simulink model "sl_pmsm"  (R2023b)
settings: Solver=VariableStepAuto  StartTime=0.0  StopTime=3  FixedStep=0.02  MaxStep=0.02  RelTol=1e-3
InitFcn:
  | init
values from neighbouring files (symbols this model uses):
  pa = block.DialogPrm(1).Data    [Animation.m]    (also in Saddle_Wave.m; current_controller.m; flux_dynamic.m; mechanical_equation.m)
libraries: spsVoltageMeasurementLib x9, simulink x4, spsSeriesRLCBranchLib x3, spsDCVoltageSourceLib x2, slpidlib x1, SignalEditorBlockLib x1, spsGroundLib x1, spsUniversalBridgeLib x1, spspowerguiLib x1
settings Model: Creator=PC  LastModifiedBy=PC

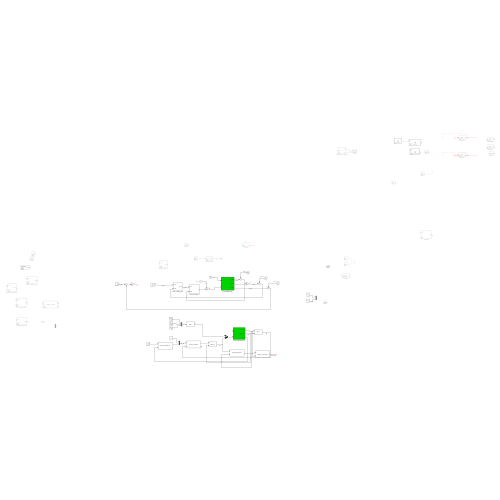
[thumbnail: Simulink's stored preview of the top-level diagram]
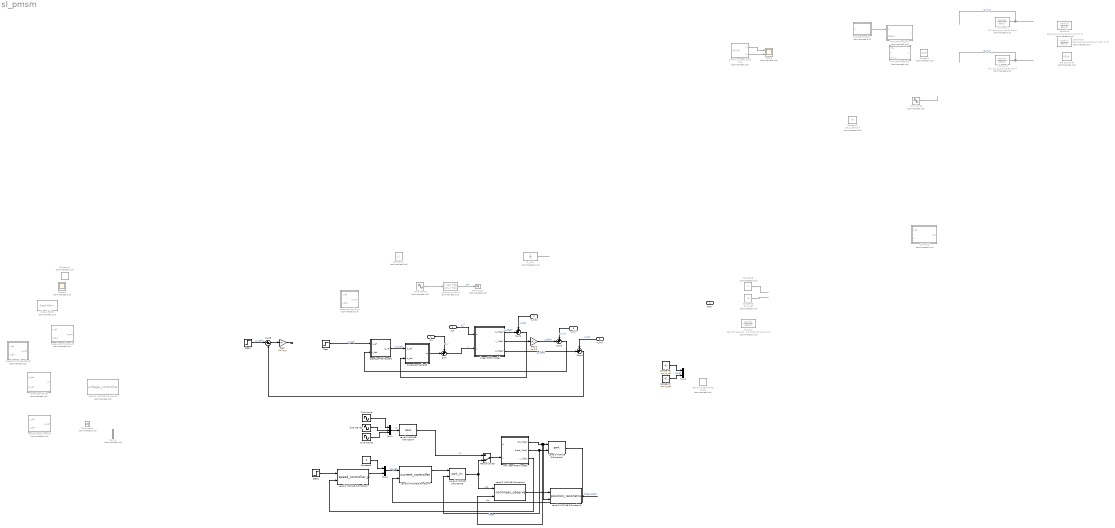
== system sl_pmsm ==
  d_v : Inport
  "n_{iq}" : Inport  Port=2
  "n_{v}" : Inport  Port=3
  d_T : Inport  Port=4
  "n_{p}" : Inport  Port=5
  Band-Limited White Noise : simulink/Sources/Band-Limited White Noise  Commented=on  Cov=[0.1]  Ts=0.1  seed=[23341]
  Constant : Constant  Commented=on  Value=pa.P
  Constant1 : Constant  Commented=on  Value=pa.iq_ref*pa.R
  Constant2 : Constant  Commented=on  Value=0.1
  Constant3 : Constant  Value=0
  Constant4 : Constant  Commented=on  Value=pa.v_ref
  Constant5 : Constant  Commented=on  Value=0
  Constant6 : Constant  Value=pa.vd_ref
  Constant7 : Constant  Value=pa.vq_ref
  Constant8 : Constant  Commented=on  Value=pa.iq_ref
  Demux : Demux  Commented=on  Outputs=2
  G_iq2w : TransferFcn  Commented=on  Denominator=[1 0]
  G_uq2w : TransferFcn  Commented=on  Numerator=[pa.Kt]  Denominator=[pa.Lq*pa.J pa.B*pa.Lq+pa.J*pa.R pa.B*pa.R+pa.Kt*pa.P/2*pa.phi_m]
  Gain : Gain  Gain=pa.Kp_p
  Gain1 : Gain  Gain=pa.P/2
  Id dynamic : TransferFcn  Commented=on  Denominator=[pa.Ls_d_H pa.Rs_Ohm]
  Iq dynamic : TransferFcn  Commented=on  Denominator=[pa.Ls_q_H pa.Rs_Ohm]
  Level-2 MATLAB S-Function1 : M-S-Function  FunctionName=speed_controller_pi  Parameters=pa
  Level-2 MATLAB S-Function2 : M-S-Function  Commented=on  FunctionName=voltage_controller  Parameters=pa
  Level-2 MATLAB S-Function3 : M-S-Function  FunctionName=nonlinear_observer  Parameters=pa
  Level-2 MATLAB S-Function4 : M-S-Function  FunctionName=current_controller  Parameters=pa
  Level-2 MATLAB S-Function5 : M-S-Function  FunctionName=park  Parameters=pa
  Level-2 MATLAB S-Function6 : M-S-Function  FunctionName=position_reconstruct  Parameters=pa
  Level-2 MATLAB S-Function7 : M-S-Function  FunctionName=clark  Parameters=pa
  Level-2 MATLAB S-Function8 : M-S-Function  FunctionName=park_inv  Parameters=pa
  MATLAB Function : MATLAB Function  Commented=on  TreatAsAtomicUnit=on
  MATLAB Function1 : MATLAB Function  Commented=on  TreatAsAtomicUnit=on
  MATLAB Function2 : MATLAB Function  Commented=on  TreatAsAtomicUnit=on
  Manual Switch : ManualSwitch  CurrentSetting=0
  Mux1 : Mux  Inputs=3
  Mux2 : Mux  Inputs=2
  Mux3 : Mux  Inputs=2
  PID Controller : slpidlib/PID Controller  Commented=on  Controller=PID  Form=Parallel  TimeDomain=Continuous-time  UseExternalTs=off  SampleTime=-1  IntegratorMethod=Forward Euler  FilterMethod=Forward Euler  ControllerParametersSource=internal  P=1  I=1  UseKiTs=off  D=0  N=100  UseFilter=on  TunerSelectOption=Transfer Function Based (PID Tuner App)  InitialConditionSource=internal  InitialConditionForIntegrator=0  InitialConditionForFilter=0  DifferentiatorICPrevScaledInput=0  ExternalReset=none  TrackingMode=off  Kt=1  LimitOutput=off  SatLimitsSource=internal  UpperSaturationLimit=inf  LowerSaturationLimit=-inf  LinearizeAsGain=on  AntiWindupMode=none  Kb=1  LimitIntegrator=off  UpperIntegratorSaturationLimit=inf  LowerIntegratorSaturationLimit=-inf  POutMin=[]  POutMax=[]  IOutMin=[]  IOutMax=[]  DOutMin=[]  DOutMax=[]  NOutMin=[]  NOutMax=[]  SumOutMin=[]  SumOutMax=[]  SaturationOutMin=[]  SaturationOutMax=[]  PParamMin=[]  PParamMax=[]  IParamMin=[]  IParamMax=[]  DParamMin=[]  DParamMax=[]  NParamMin=[]  NParamMax=[]  KbParamMin=[]  KbParamMax=[]  KtParamMin=[]  KtParamMax=[]  KbOutMin=[]  KbOutMax=[]  KtOutMin=[]  KtOutMax=[]  IntegratorOutMin=[]  IntegratorOutMax=[]  FilterOutMin=[]  FilterOutMax=[]  SumI1OutMin=[]  SumI1OutMax=[]  SumI2OutMin=[]  SumI2OutMax=[]  SumI3OutMin=[]  SumI3OutMax=[]  SumI4OutMin=[]  SumI4OutMax=[]  SumDOutMin=[]  SumDOutMax=[]  DifferentiatorOutMin=[]  DifferentiatorOutMax=[]  FilterDiffOutCoefMin=[]  FilterDiffOutCoefMax=[]  ReciprocalOutMin=[]  ReciprocalOutMax=[]  SumDenOutMin=[]  SumDenOutMax=[]  SumNumOutMin=[]  SumNumOutMax=[]  DivideOutMin=[]  DivideOutMax=[]  UdiffTsProdOutMin=[]  UdiffTsProdOutMax=[]  NTsProdOutMin=[]  NTsProdOutMax=[]  UintegralTsProdOutMin=[]  UintegralTsProdOutMax=[]  UngainTsProdOutMin=[]  UngainTsProdOutMax=[]  ClampingZeroOutDataTypeStr=Inherit: Inherit via back propagation  ClampingZeroOutMin=[]  ClampingZeroOutMax=[]  FilterDenConstantOutDataTypeStr=Inherit: Inherit via back propagation  FilterDenConstantOutMin=[]  FilterDenConstantOutMax=[]  PCopyOutDataTypeStr=Inherit: Inherit via back propagation  PCopyOutMin=[]  PCopyOutMax=[]  NCopyOutDataTypeStr=Inherit: Inherit via back propagation  NCopyOutMin=[]  NCopyOutMax=[]  IntegratorContinuousStateAttributes=''  IntegratorStateMustResolveToSignalObject=off  IntegratorRTWStateStorageClass=Auto  FilterContinuousStateAttributes=''  FilterStateMustResolveToSignalObject=off  FilterRTWStateStorageClass=Auto  ParallelPVariant=InternalParameters  IdealPVariant=Disabled  IVariant=InternalParameters  DVariant=InternalParameters  IntegratorVariant=Continuous  SatVariant=Disabled  AWVariant=Passthrough  PCopyVariant=Disabled  TRVariant=Disabled  FdbkBlocksVariant=Forward  IdealPFdbkVariant=Disabled  SatFdbkVariant=Disabled  DerivativeFilterVariant=ContFilter  NVariant=InternalParameters  NCopyVariant=Disabled  FilterICVariant=InternalICsFilter  IntegratorICVariant=InternalICs  ExternalResetVariant=Disabled  TRSumVariant=Passthrough  SumFdbkVariant=Disabled  SumVariant=Sum_PID  TsampFilterVariant=InternalTs  TsampNgainVariant=Passthrough  TsampIntegralVariant=Disabled_SignalSpec  ExternalSaturationOutDataTypeStr=Inherit: Same as second input
  Scope : Scope  Commented=on  NumInputPorts=2
  Scope1 : Scope  Commented=on
  Signal Editor : SignalEditorBlockLib/Signal Editor  Commented=on  FileName=ramp.mat  ActiveScenario=Scenario  ActiveSignal=Signal 1  IsBus=off  OutputBusObjectStr=Bus: BusObject  SampleTime=0  Interpolate=off  ZeroCross=off  OutputAfterFinalValue=Holding final value  Unit=inherit  PreserveSignalName=on  ApplySigPropsToAllScenarios=on  ApplySigPropsToAllSignals=off
  Sine Wave : Sin  Frequency=50*2*pi  SampleTime=0
  Sine Wave1 : Sin  Frequency=50*2*pi  Phase=-2*pi/3  SampleTime=0
  Sine Wave2 : Sin  Frequency=50*2*pi  Phase=2*pi/3  SampleTime=0
  Sine Wave3 : Sin  Commented=on  Amplitude=1.0  Frequency=1*2*pi  SampleTime=0
  Sine Wave4 : Sin  Commented=on  Frequency=50*2*pi  Phase=-pi/2  SampleTime=0
  Step : Step  After=pa.v_ref  SampleTime=0
  Step1 : Step  After=pa.v_ref  SampleTime=0
  Step2 : Step  After=pa.p_vef  SampleTime=0
  Sum{,1..2,4} (4 alike) : Sum  Inputs=++|
  Sum3 : Sum  Inputs=|+-
  Terminator : Terminator  Commented=on
  Terminator1 : Terminator  Commented=on
  controller : TransferFcn  Commented=on  Numerator=[pa.Kp_Iq pa.Kp_Iq*pa.Ki_Iq]  Denominator=[1 0]
  controller1 : TransferFcn  Commented=on  Numerator=[pa.Kp_Id pa.Kp_Id*pa.Ki_Id]  Denominator=[1 0]
  controller_polynomial : Subsystem  Commented=on
  current_controller : Subsystem  Commented=on
  current_controller_tf : Subsystem
  dq model : Subsystem  Commented=on
  linear PMSM model : Subsystem
  nonlinear PMSM model : Subsystem
  simplify current close loop : Subsystem  Commented=on
  speed_controller_adrc : Subsystem
  speed_controller_adrc_tf : Subsystem  Commented=on
  speed_controller_pi : Subsystem  Commented=on
  speed_controller_pi_tf : Subsystem  Commented=on
  velocity dynamic : StateSpace  Commented=on  A=-0.5  B=1058  D=0  InitialCondition=0
  error : Outport
  wires:
  Iq dynamic/1 -> ?  "Iq_in_A"
  Id dynamic/1 -> ?  "Id_in_A"
  ? -> Id dynamic/1
  Step1/1 -> Level-2 MATLAB S-Function1/1
  ? -> Iq dynamic/1
  MATLAB Function/1(y) -> MATLAB Function1/1(u)
  Sine Wave/1 -> Mux1/1
  Sine Wave1/1 -> Mux1/2
  Sine Wave2/1 -> Mux1/3
  Mux1/1 -> Level-2 MATLAB S-Function7/1  "v1"
  Sine Wave4/1 -> ?
  Level-2 MATLAB S-Function7/1 -> Manual Switch/1  "v2"
  simplify current close loop/1(id) -> Scope/1
  simplify current close loop/2(iq) -> Scope/2
  Sine Wave3/1 -> velocity dynamic/1
  velocity dynamic/1 -> Terminator/1  "v_ol"
  Constant7/1 -> Mux2/2  "vq_ref"
  Constant6/1 -> Mux2/1
  current_controller_tf/1(uq) -> Sum/2
  d_v/1 -> Sum/1  "d_v"
  "n_{v}"/1 -> Sum2/1  "n_{v}"
  speed_controller_adrc/1(iq_ref) -> current_controller_tf/1(iq_ref)  "iq_{ref}"
  Constant8/1 -> ?
  Constant5/1 -> ?
  Constant3/1 -> Mux3/1
  Mux3/1 -> Level-2 MATLAB S-Function4/1  "idq_ref"
  Level-2 MATLAB S-Function1/1 -> Mux3/2
  Step2/1 -> Sum3/1  "p_{ref}"
  Sum3/1 -> Gain/1
  "n_{iq}"/1 -> Sum1/1  "n_{iq}"
  Sum1/1 -> current_controller_tf/2(iq_fed)
  d_T/1 -> linear PMSM model/1(d)  "d_T"
  Sum/1 -> linear PMSM model/2(u)  "u"
  linear PMSM model/1("iq_{fed}") -> Sum1/2  "iq_{fed}"
  linear PMSM model/2("v_{fed}") -> Gain1/1
  Manual Switch/1 -> nonlinear PMSM model/2(u)
  linear PMSM model/3("p_{fed}") -> Sum4/2  "p_{fed}"
  "n_{p}"/1 -> Sum4/1  "n_{p}"
  Step/1 -> speed_controller_adrc/1(v_ref)  "v_{ref}"
  Sum2/1 -> speed_controller_adrc/2(v_fed)
  Sum4/1 -> Sum3/2
  Gain/1 -> ?
  Gain1/1 -> Sum2/2  "v_{fed}"
  G_iq2w/1 -> ?
  nonlinear PMSM model/1("Iab_{fed}") -> Level-2 MATLAB S-Function6/2, Level-2 MATLAB S-Function5/1, Level-2 MATLAB S-Function3/2
  nonlinear PMSM model/2("theta_{fed}") -> Level-2 MATLAB S-Function8/2, Level-2 MATLAB S-Function5/2  "theta"
  Level-2 MATLAB S-Function5/1 -> Level-2 MATLAB S-Function4/2  "idq"
  nonlinear PMSM model/3("v_{fed}") -> Level-2 MATLAB S-Function1/2
  Level-2 MATLAB S-Function4/1 -> Level-2 MATLAB S-Function8/1
  Level-2 MATLAB S-Function8/1 -> Manual Switch/2, Level-2 MATLAB S-Function3/1  "vab"
  Level-2 MATLAB S-Function3/1 -> Level-2 MATLAB S-Function6/1
  Level-2 MATLAB S-Function6/1 -> ?  "theta_{hat}"

== system sl_pmsm/controller_polynomial ==
  v_ref : Inport
  v_fed : Inport  Port=2
  C_polynomial : TransferFcn  Numerator=[1 1]  Denominator=[1 1]
  Sum4 : Sum  Inputs=|+-
  iq_ref : Outport
  wires:
  C_polynomial/1 -> iq_ref/1
  Sum4/1 -> C_polynomial/1
  v_fed/1 -> Sum4/2
  v_ref/1 -> Sum4/1

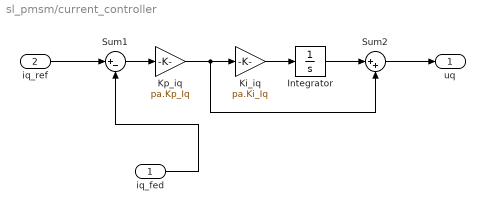
== system sl_pmsm/current_controller ==
  iq_fed : Inport
  iq_ref : Inport  Port=2
  Integrator : Integrator
  Ki_iq : Gain  Gain=pa.Ki_Iq
  Kp_iq : Gain  Gain=pa.Kp_Iq
  Sum1 : Sum  Inputs=|+-
  Sum2 : Sum  Inputs=|++
  uq : Outport
  wires:
  Ki_iq/1 -> Integrator/1
  Sum1/1 -> Kp_iq/1
  Integrator/1 -> Sum2/1
  Kp_iq/1 -> Sum2/2, Ki_iq/1
  iq_fed/1 -> Sum1/2
  iq_ref/1 -> Sum1/1
  Sum2/1 -> uq/1

== system sl_pmsm/current_controller_tf ==
  iq_ref : Inport
  iq_fed : Inport  Port=2
  C_i : TransferFcn  Numerator=[pa.Kp_Iq pa.Kp_Iq*pa.Ki_Iq]  Denominator=[1 0]
  C_i_gen : TransferFcn  Numerator=[1 1]  Denominator=[1 1]
  Sum1 : Sum  Inputs=|+-
  uq : Outport
  wires:
  iq_ref/1 -> Sum1/1
  iq_fed/1 -> Sum1/2
  Sum1/1 -> C_i/1
  C_i/1 -> uq/1

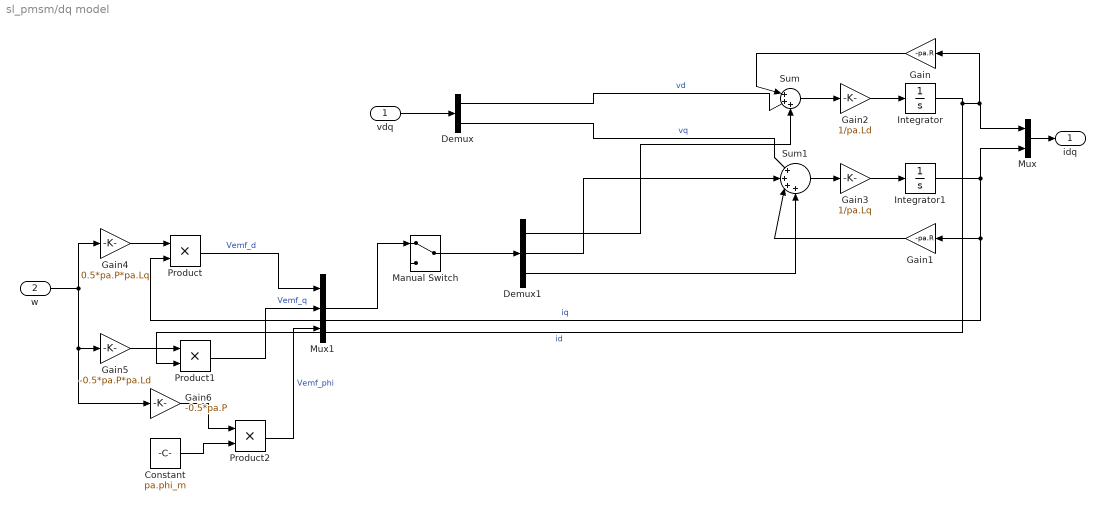
== system sl_pmsm/dq model ==
  vdq : Inport
  w : Inport  Port=2
  Constant : Constant  Value=pa.phi_m
  Demux : Demux  Outputs=2
  Demux1 : Demux  Outputs=3
  Gain : Gain  Gain=-pa.R
  Gain1 : Gain  Gain=-pa.R
  Gain2 : Gain  Gain=1/pa.Ld
  Gain3 : Gain  Gain=1/pa.Lq
  Gain4 : Gain  Gain=0.5*pa.P*pa.Lq
  Gain5 : Gain  Gain=-0.5*pa.P*pa.Ld
  Gain6 : Gain  Gain=-0.5*pa.P
  Integrator : Integrator
  Integrator1 : Integrator
  Manual Switch : ManualSwitch
  Mux : Mux  Inputs=2
  Mux1 : Mux  Inputs=3
  Product : Product
  Product1 : Product
  Product2 : Product
  Sum : Sum  Inputs=|+++
  Sum1 : Sum  Inputs=|++++
  idq : Outport
  wires:
  Mux/1 -> idq/1
  Integrator/1 -> Product1/2, Gain/1, Mux/1  "id"
  Integrator1/1 -> Mux/2, Gain1/1, Product/2  "iq"
  vdq/1 -> Demux/1
  Sum/1 -> Gain2/1
  Sum1/1 -> Gain3/1
  Demux/1 -> Sum/2  "vd"
  Demux/2 -> Sum1/1  "vq"
  w/1 -> Gain4/1, Gain6/1, Gain5/1
  Gain4/1 -> Product/1
  Gain5/1 -> Product1/1
  Gain6/1 -> Product2/1
  Constant/1 -> Product2/2
  Gain/1 -> Sum/1
  Gain1/1 -> Sum1/3
  Gain2/1 -> Integrator/1
  Gain3/1 -> Integrator1/1
  Demux1/1 -> Sum/3
  Product/1 -> Mux1/1  "Vemf_d"
  Demux1/2 -> Sum1/2
  Product1/1 -> Mux1/2  "Vemf_q"
  Demux1/3 -> Sum1/4
  Product2/1 -> Mux1/3  "Vemf_phi"
  Manual Switch/1 -> Demux1/1
  Mux1/1 -> Manual Switch/1

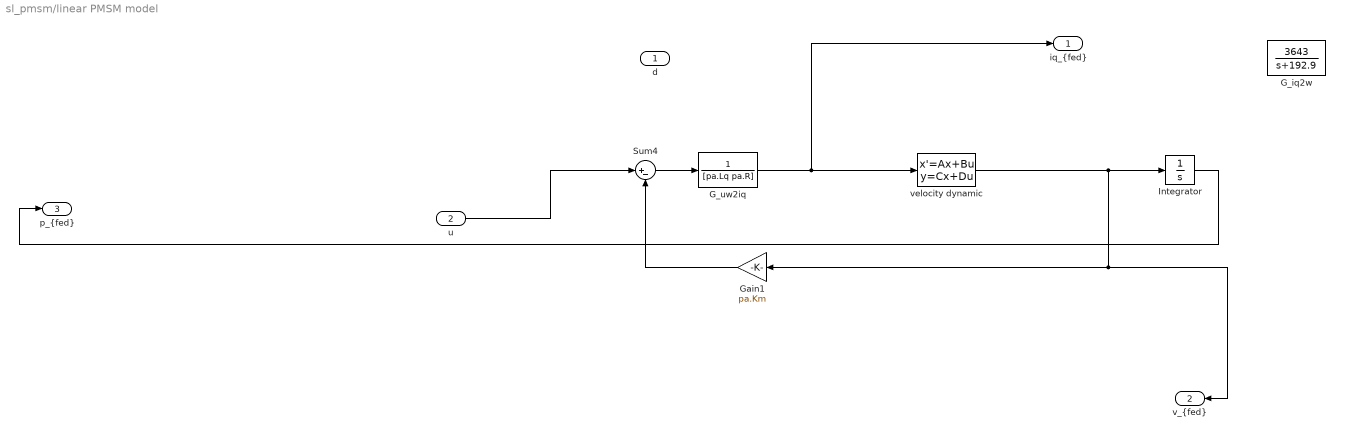
== system sl_pmsm/linear PMSM model ==
  d : Inport
  u : Inport  Port=2
  G_iq2w : TransferFcn  Numerator=[3643]  Denominator=[1 192.9]
  G_uw2iq : TransferFcn  Denominator=[pa.Lq pa.R]
  Gain1 : Gain  Gain=pa.Km
  Integrator : Integrator
  Sum4 : Sum  Inputs=|+-
  velocity dynamic : StateSpace  A=-0.5  B=1058  D=0  InitialCondition=0
  "iq_{fed}" : Outport
  "v_{fed}" : Outport  Port=2
  "p_{fed}" : Outport  Port=3
  wires:
  u/1 -> Sum4/1
  velocity dynamic/1 -> Integrator/1, "v_{fed}"/1, Gain1/1
  Gain1/1 -> Sum4/2
  Sum4/1 -> G_uw2iq/1
  G_uw2iq/1 -> velocity dynamic/1, "iq_{fed}"/1
  Integrator/1 -> "p_{fed}"/1

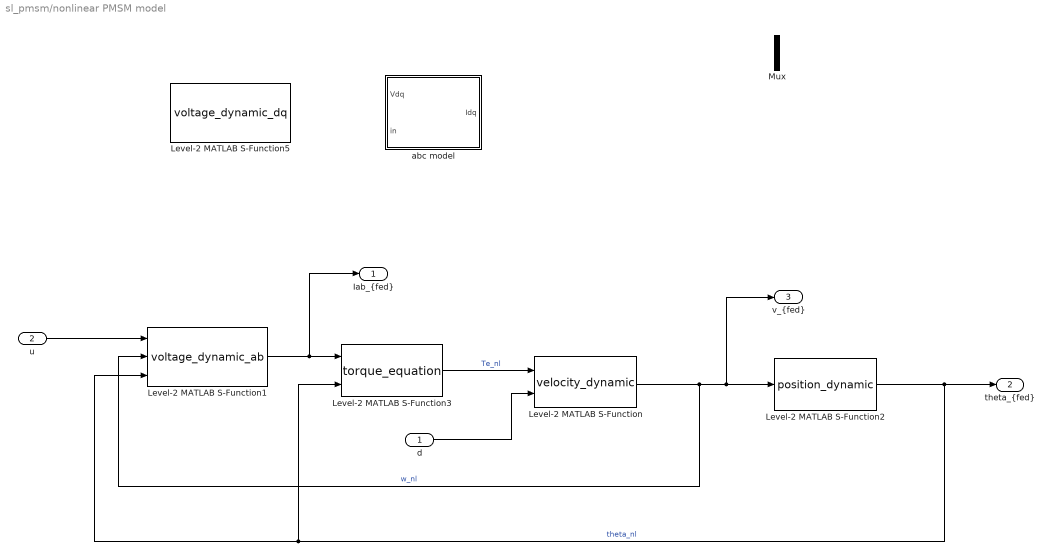
== system sl_pmsm/nonlinear PMSM model ==
  d : Inport
  u : Inport  Port=2
  Level-2 MATLAB S-Function : M-S-Function  FunctionName=velocity_dynamic  Parameters=pa
  Level-2 MATLAB S-Function1 : M-S-Function  FunctionName=voltage_dynamic_ab  Parameters=pa
  Level-2 MATLAB S-Function2 : M-S-Function  FunctionName=position_dynamic  Parameters=pa
  Level-2 MATLAB S-Function3 : M-S-Function  FunctionName=torque_equation  Parameters=pa
  Level-2 MATLAB S-Function5 : M-S-Function  FunctionName=voltage_dynamic_dq  Parameters=pa
  Mux : Mux  Inputs=2
  abc model : Subsystem
  "Iab_{fed}" : Outport
  "theta_{fed}" : Outport  Port=2
  "v_{fed}" : Outport  Port=3
  wires:
  Level-2 MATLAB S-Function3/1 -> Level-2 MATLAB S-Function/1  "Te_nl"
  Level-2 MATLAB S-Function/1 -> Level-2 MATLAB S-Function2/1, "v_{fed}"/1, Level-2 MATLAB S-Function1/2  "w_nl"
  Level-2 MATLAB S-Function2/1 -> "theta_{fed}"/1, Level-2 MATLAB S-Function3/2, Level-2 MATLAB S-Function1/3  "theta_nl"
  d/1 -> Level-2 MATLAB S-Function/2
  u/1 -> Level-2 MATLAB S-Function1/1
  Level-2 MATLAB S-Function1/1 -> "Iab_{fed}"/1, Level-2 MATLAB S-Function3/1

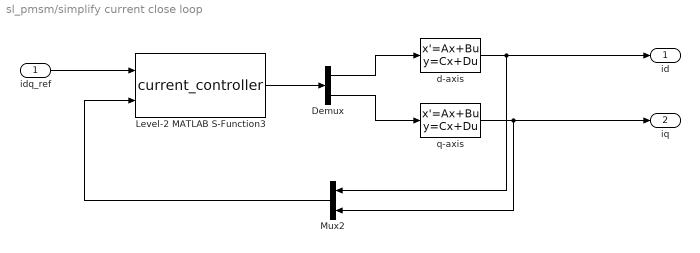
== system sl_pmsm/simplify current close loop ==
  idq_ref : Inport
  Demux : Demux  Outputs=2
  Level-2 MATLAB S-Function3 : M-S-Function  FunctionName=current_controller  Parameters=pa
  Mux2 : Mux  Inputs=2
  d-axis : StateSpace  A=-pa.R/pa.Ld  B=1/pa.Ld  D=0  InitialCondition=0
  q-axis : StateSpace  A=-pa.R/pa.Lq  B=1/pa.Lq  D=0  InitialCondition=0
  id : Outport
  iq : Outport  Port=2
  wires:
  Demux/2 -> q-axis/1
  d-axis/1 -> id/1, Mux2/1
  Mux2/1 -> Level-2 MATLAB S-Function3/2
  Level-2 MATLAB S-Function3/1 -> Demux/1
  q-axis/1 -> iq/1, Mux2/2
  Demux/1 -> d-axis/1
  idq_ref/1 -> Level-2 MATLAB S-Function3/1

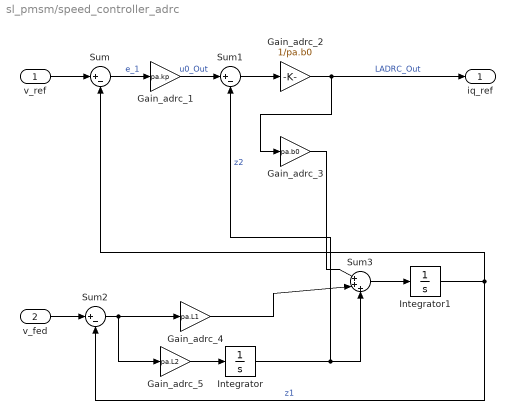
== system sl_pmsm/speed_controller_adrc ==
  v_ref : Inport
  v_fed : Inport  Port=2
  Gain_adrc_1 : Gain  Gain=pa.kp
  Gain_adrc_2 : Gain  Gain=1/pa.b0
  Gain_adrc_3 : Gain  Gain=pa.b0
  Gain_adrc_4 : Gain  Gain=pa.L1
  Gain_adrc_5 : Gain  Gain=pa.L2
  Integrator : Integrator
  Integrator1 : Integrator
  Sum : Sum  Inputs=|+-
  Sum1 : Sum  Inputs=|+-
  Sum2 : Sum  Inputs=|+-
  Sum3 : Sum  Inputs=|+++
  iq_ref : Outport
  wires:
  Gain_adrc_2/1 -> iq_ref/1, Gain_adrc_3/1  "LADRC_Out"
  Sum3/1 -> Integrator1/1
  Gain_adrc_4/1 -> Sum3/2
  Integrator/1 -> Sum3/3, Sum1/2  "z2"
  Sum2/1 -> Gain_adrc_5/1, Gain_adrc_4/1
  Sum1/1 -> Gain_adrc_2/1
  Integrator1/1 -> Sum2/2, Sum/2  "z1"
  Sum/1 -> Gain_adrc_1/1  "e_1"
  Gain_adrc_3/1 -> Sum3/1
  Gain_adrc_5/1 -> Integrator/1
  Gain_adrc_1/1 -> Sum1/1  "u0_Out"
  v_ref/1 -> Sum/1
  v_fed/1 -> Sum2/1

== system sl_pmsm/speed_controller_adrc_tf ==
  v_ref : Inport
  v_fed : Inport  Port=2
  C : TransferFcn  Numerator=[pa.beta1*pa.l1+pa.beta2 pa.beta2*pa.l1]  Denominator=pa.b0*[1 pa.beta1+pa.l1 0]
  C1 : TransferFcn  Numerator=pa.l1*[1 pa.beta1 pa.beta2]  Denominator=[1 pa.beta1*pa.l1+pa.beta2 pa.beta2*pa.l1]
  Sum : Sum  Inputs=|+-
  iq_ref : Outport
  wires:
  v_ref/1 -> C1/1
  C1/1 -> Sum/1
  v_fed/1 -> Sum/2
  Sum/1 -> C/1
  C/1 -> iq_ref/1

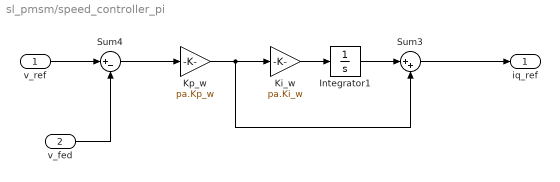
== system sl_pmsm/speed_controller_pi ==
  v_ref : Inport
  v_fed : Inport  Port=2
  Integrator1 : Integrator
  Ki_w : Gain  Gain=pa.Ki_w
  Kp_w : Gain  Gain=pa.Kp_w
  Sum3 : Sum  Inputs=|++
  Sum4 : Sum  Inputs=|+-
  iq_ref : Outport
  wires:
  Sum4/1 -> Kp_w/1
  v_fed/1 -> Sum4/2
  Kp_w/1 -> Ki_w/1, Sum3/2
  Ki_w/1 -> Integrator1/1
  Integrator1/1 -> Sum3/1
  Sum3/1 -> iq_ref/1
  v_ref/1 -> Sum4/1

== system sl_pmsm/speed_controller_pi_tf ==
  v_ref : Inport
  v_fed : Inport  Port=2
  C_v : TransferFcn  Numerator=[pa.Kp_v pa.Kp_v*pa.Ki_v]  Denominator=[1 0]
  C_v_gen : TransferFcn  Numerator=[1 1]  Denominator=[1 1]
  Sum4 : Sum  Inputs=|+-
  iq_ref : Outport
  wires:
  v_ref/1 -> Sum4/1
  v_fed/1 -> Sum4/2
  Sum4/1 -> C_v/1
  C_v/1 -> iq_ref/1

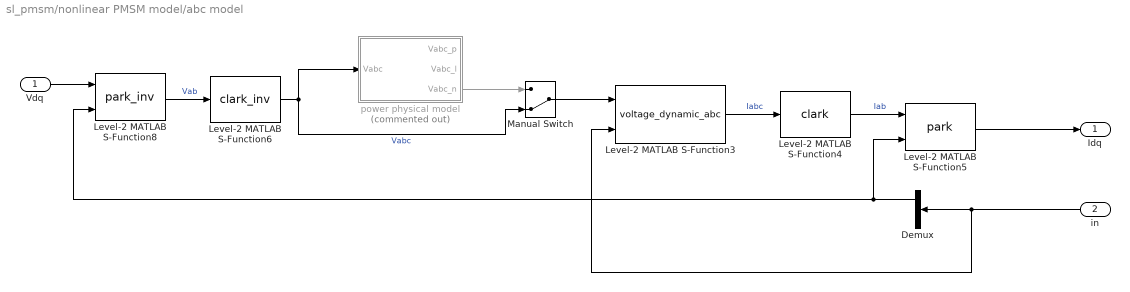
== system sl_pmsm/nonlinear PMSM model/abc model ==
  Vdq : Inport
  in : Inport  Port=2
  Demux : Demux  Outputs=2
  Level-2 MATLAB S-Function3 : M-S-Function  FunctionName=voltage_dynamic_abc  Parameters=pa
  Level-2 MATLAB S-Function4 : M-S-Function  FunctionName=clark  Parameters=pa
  Level-2 MATLAB S-Function5 : M-S-Function  FunctionName=park  Parameters=pa
  Level-2 MATLAB S-Function6 : M-S-Function  FunctionName=clark_inv  Parameters=pa
  Level-2 MATLAB S-Function8 : M-S-Function  FunctionName=park_inv  Parameters=pa
  Manual Switch : ManualSwitch  CurrentSetting=0
  power physical model : Subsystem  Commented=on
  Idq : Outport
  wires:
  Level-2 MATLAB S-Function6/1 -> power physical model/1(Vabc), Manual Switch/2  "Vabc"
  Level-2 MATLAB S-Function8/1 -> Level-2 MATLAB S-Function6/1  "Vab"
  Level-2 MATLAB S-Function4/1 -> Level-2 MATLAB S-Function5/1  "Iab"
  Level-2 MATLAB S-Function3/1 -> Level-2 MATLAB S-Function4/1  "Iabc"
  Vdq/1 -> Level-2 MATLAB S-Function8/1
  Manual Switch/1 -> Level-2 MATLAB S-Function3/1
  power physical model/3(Vabc_n) -> Manual Switch/1
  Level-2 MATLAB S-Function5/1 -> Idq/1
  in/1 -> Level-2 MATLAB S-Function3/2, Demux/1
  Demux/1 -> Level-2 MATLAB S-Function8/2, Level-2 MATLAB S-Function5/2

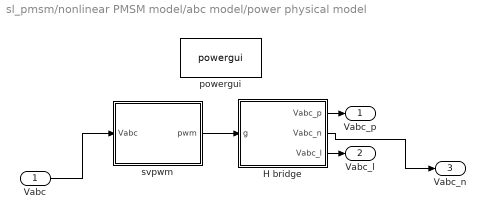
== system sl_pmsm/nonlinear PMSM model/abc model/power physical model ==
  Vabc : Inport
  "H bridge " : Subsystem
  powergui : spspowerguiLib/powergui  Priority=1  SimulationMode=Continuous  SampleTime=50e-6  frequency=60  Iterations=50  frequencyindice=0  Pbase=100e6  ErrMax=1e-4  UnitsV=kV  UnitsW=MW  buscounter=0  FunctionMessages=off  echomessages=off  EnableUseOfTLC=off  CurrentSourceSwitches=off  DisableSnubberDevices=off  DisableRonSwitches=off  DisableVfSwitches=off  DisplayEquations=off  AutomaticDiscreteSolvers=off  SolverType=Tustin/Backward Euler (TBE)  Interpol=off  ExternalGateDelay=off  methode=off  Ts=100  x0status=blocks  SPID=on  SwTol=0  HookPort=off  NonlinearTolerance=1e-4  nMaxIteration=100  ContinueOnMaxIteration=off  RestoreLinks=warning  ResistiveCurrentMeasurement=off  Frange=[0:2:500]  Ylog=off  Xlog=on  ShowGrid=off  save=off  variable=ZData  structure=0  ZoomFFT=off  StartTime=0.0  cycles=1  DisplayStyle=1  fundamental=60  FreqAxis=off  MaxFrequency=1000  frequencyindicesteady=1  RmsSteady=1  display=off
  svpwm : Subsystem
  Vabc_p : Outport
  Vabc_l : Outport  Port=2
  Vabc_n : Outport  Port=3
  wires:
  svpwm/1(pwm) -> "H bridge "/1(g)
  "H bridge "/2(Vabc_n) -> Vabc_n/1
  "H bridge "/1(Vabc_p) -> Vabc_p/1
  Vabc/1 -> svpwm/1(Vabc)
  "H bridge "/3(Vabc_l) -> Vabc_l/1

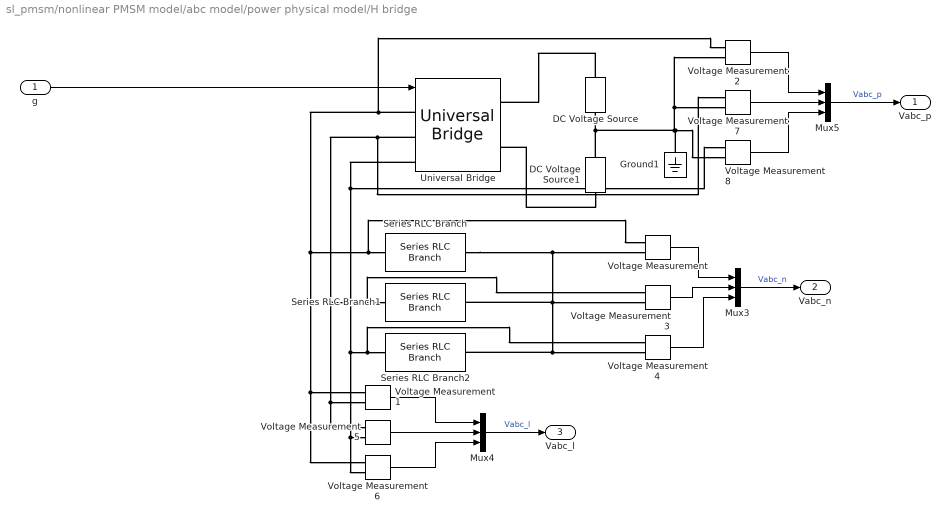
== system sl_pmsm/nonlinear PMSM model/abc model/power physical model/H bridge  ==
  g : Inport
  DC Voltage Source : spsDCVoltageSourceLib/DC Voltage Source  Amplitude=pa.dc/2  Measurements=None
  DC Voltage Source1 : spsDCVoltageSourceLib/DC Voltage Source  Amplitude=pa.dc/2  Measurements=None
  Ground1 : spsGroundLib/Ground  LConnTagsString=a
  Mux3 : Mux  Inputs=3
  Mux4 : Mux  Inputs=3
  Mux5 : Mux  Inputs=3
  Series RLC Branch : spsSeriesRLCBranchLib/Series RLC Branch  LConnTagsString=__new0  RConnTagsString=__new0  BranchType=RL  Resistance=1  Inductance=1e-3  SetiL0=off  InitialCurrent=0  Capacitance=1e-6  Setx0=off  InitialVoltage=0  Measurements=None
  Series RLC Branch1 : spsSeriesRLCBranchLib/Series RLC Branch  LConnTagsString=__new0  RConnTagsString=__new0  BranchType=RL  Resistance=1  Inductance=1e-3  SetiL0=off  InitialCurrent=0  Capacitance=1e-6  Setx0=off  InitialVoltage=0  Measurements=None
  Series RLC Branch2 : spsSeriesRLCBranchLib/Series RLC Branch  LConnTagsString=__new0  RConnTagsString=__new0  BranchType=RL  Resistance=1  Inductance=1e-3  SetiL0=off  InitialCurrent=0  Capacitance=1e-6  Setx0=off  InitialVoltage=0  Measurements=None
  Universal Bridge : spsUniversalBridgeLib/Universal Bridge  Arms=3  SnubberResistance=1e5  SnubberCapacitance=inf  Device=MOSFET / Diodes  Ron=1e-3  Lon=0  ForwardVoltages="[  0  0  ]"  ForwardVoltage=0  GTOparameters=[ 10e-6 , 20e-6 ]  IGBTparameters=[ 1e-6 , 2e-6 ]  Measurements=None  Measurements_2=None  converterType=Rectifier
  Voltage Measurement{,1..8} (9 alike) : spsVoltageMeasurementLib/Voltage Measurement  PhasorSimulation=off  OutputType=Complex  PSBequivalent=0
  Vabc_p : Outport
  Vabc_n : Outport  Port=2
  Vabc_l : Outport  Port=3
  wires:
  Voltage Measurement2/1 -> Mux5/1
  Voltage Measurement1/1 -> Mux4/1
  Voltage Measurement/1 -> Mux3/1
  Voltage Measurement6/1 -> Mux4/3
  Voltage Measurement3/1 -> Mux3/2
  Voltage Measurement8/1 -> Mux5/3
  Voltage Measurement4/1 -> Mux3/3
  Voltage Measurement7/1 -> Mux5/2
  Voltage Measurement5/1 -> Mux4/2
  Mux5/1 -> Vabc_p/1  "Vabc_p"
  Mux4/1 -> Vabc_l/1  "Vabc_l"
  Mux3/1 -> Vabc_n/1  "Vabc_n"
  g/1 -> Universal Bridge/1
  connections:
  Universal Bridge/LConn3 -- Voltage Measurement8/LConn1 -- Voltage Measurement6/LConn2 -- Voltage Measurement5/LConn2 -- Voltage Measurement4/LConn1 -- Series RLC Branch2/LConn1
  Universal Bridge/LConn1 -- Voltage Measurement2/LConn1 -- Voltage Measurement6/LConn1 -- Voltage Measurement1/LConn1 -- Voltage Measurement/LConn1 -- Series RLC Branch/LConn1
  Universal Bridge/LConn2 -- Voltage Measurement7/LConn1 -- Voltage Measurement1/LConn2 -- Voltage Measurement5/LConn1 -- Voltage Measurement3/LConn1 -- Series RLC Branch1/LConn1
  DC Voltage Source1/RConn1 -- Ground1/LConn1 -- Voltage Measurement8/LConn2 -- Voltage Measurement7/LConn2 -- Voltage Measurement2/LConn2 -- DC Voltage Source/LConn1
  DC Voltage Source/RConn1 -- Universal Bridge/RConn1
  DC Voltage Source1/LConn1 -- Universal Bridge/RConn2
  Series RLC Branch/RConn1 -- Voltage Measurement3/LConn2 -- Series RLC Branch1/RConn1 -- Series RLC Branch2/RConn1 -- Voltage Measurement4/LConn2 -- Voltage Measurement/LConn2

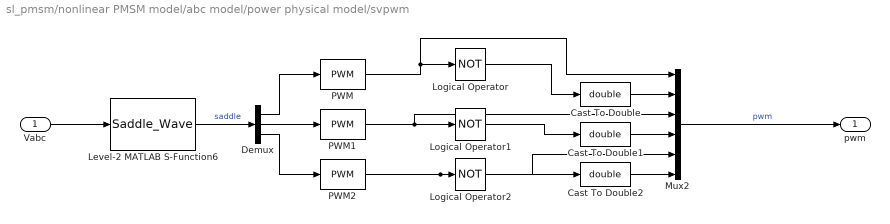
== system sl_pmsm/nonlinear PMSM model/abc model/power physical model/svpwm ==
  Vabc : Inport
  Cast To Double : DataTypeConversion  OutDataTypeStr=double  SaturateOnIntegerOverflow=off  RndMeth=Floor
  Cast To Double1 : DataTypeConversion  OutDataTypeStr=double  SaturateOnIntegerOverflow=off  RndMeth=Floor
  Cast To Double2 : DataTypeConversion  OutDataTypeStr=double  SaturateOnIntegerOverflow=off  RndMeth=Floor
  Demux : Demux  Outputs=3
  Level-2 MATLAB S-Function6 : M-S-Function  FunctionName=Saddle_Wave  Parameters=pa
  Logical Operator : Logic  Operator=NOT  AllPortsSameDT=off  OutDataTypeStr=boolean
  Logical Operator1 : Logic  Operator=NOT  AllPortsSameDT=off  OutDataTypeStr=boolean
  Logical Operator2 : Logic  Operator=NOT  AllPortsSameDT=off  OutDataTypeStr=boolean
  Mux2 : Mux  Inputs=6
  PWM : simulink/Discontinuities/PWM  DisableCoverage=on  Period=1/(pa.CarrFreq*1000)  InitialDelay=0  DisallowZeroDutyCycle=off  RunAtFixedTimeIntervals=off  SampleTime=0.1
  PWM1 : simulink/Discontinuities/PWM  DisableCoverage=on  Period=1/(pa.CarrFreq*1000)  InitialDelay=0  DisallowZeroDutyCycle=off  RunAtFixedTimeIntervals=off  SampleTime=0.1
  PWM2 : simulink/Discontinuities/PWM  DisableCoverage=on  Period=1/(pa.CarrFreq*1000)  InitialDelay=0  DisallowZeroDutyCycle=off  RunAtFixedTimeIntervals=off  SampleTime=0.1
  pwm : Outport
  wires:
  PWM1/1 -> Logical Operator1/1, Mux2/3
  Logical Operator/1 -> Cast To Double/1
  Mux2/1 -> pwm/1  "pwm"
  Vabc/1 -> Level-2 MATLAB S-Function6/1
  PWM/1 -> Mux2/1, Logical Operator/1
  Logical Operator2/1 -> Cast To Double2/1
  Demux/2 -> PWM1/1
  Demux/1 -> PWM/1
  Cast To Double2/1 -> Mux2/6
  PWM2/1 -> Mux2/5, Logical Operator2/1
  Level-2 MATLAB S-Function6/1 -> Demux/1  "saddle"
  Cast To Double/1 -> Mux2/2
  Logical Operator1/1 -> Cast To Double1/1
  Demux/3 -> PWM2/1
  Cast To Double1/1 -> Mux2/4

== matlab function sl_pmsm/MATLAB Function1 ==
  data: u input; y output; theta_r input; pa data_store_memory
function y = park_tf(u,theta_r)
global pa;
P = pa.P;
theta_e = P/2 * theta_r;
park = [cos(theta_e) sin(theta_e);
        -sin(theta_e) cos(theta_e)];
y = park*u;

== matlab function sl_pmsm/MATLAB Function ==
  data: u input; y output
function y = clark_tf(u)
clark = 2/3 * [1 -1/2 -1/2;
               0 sqrt(3)/2 -sqrt(3)/2];
y = clark*u;

== matlab function sl_pmsm/MATLAB Function2 ==
  data: idq input; y output; P input; phi_m input
function y = torque_equation(idq,P,phi_m)

ied = idq(1);
ieq = idq(2);

phi_m = pa.phi_m;
P = pa.P;

% Te = 3*P/4 *(phi_m*ieq - (Lq-Ld)*ied*ieq);
Te = 3*P/4 *(phi_m*ieq);

y = Te;
